simulink model "model_1"  (R2017a)
settings: Solver=VariableStepAuto  StartTime=0.0  StopTime=200000  FixedStep=0.0001  RelTol=1e-6
values from neighbouring files (symbols this model uses):
  c = 3    [Zbiornik.m]
  F_C = Fc0    (= 27)    [Zbiornik.m]
  F_D = Fd0    (= 12)    [Zbiornik.m]
  F_H = Fh0    (= 15)    [Zbiornik.m]
settings Model: Creator=dq  LastModifiedBy=dq

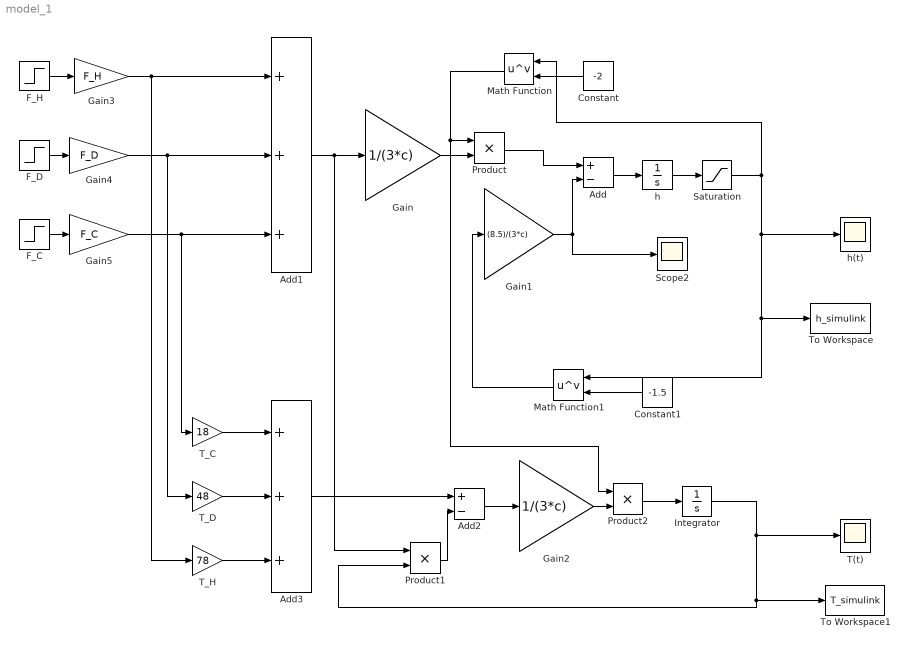
== system model_1 ==
  Add : Sum  Inputs=+-
  Add1 : Sum  Inputs=+++
  Add2 : Sum  Inputs=+-
  Add3 : Sum  Inputs=+++
  Constant : Constant  Value=-2
  Constant1 : Constant  Value=-1.5
  F_C : Step  SampleTime=0
  F_D : Step  SampleTime=0
  F_H : Step  SampleTime=0
  Gain : Gain  Gain=1/(3*c)
  Gain1 : Gain  Gain=(8.5)/(3*c)
  Gain2 : Gain  Gain=1/(3*c)
  Gain3 : Gain  Gain=F_H
  Gain4 : Gain  Gain=F_D
  Gain5 : Gain  Gain=F_C
  Integrator : Integrator
  Math Function : Math  Operator=pow  OutputSignalType=real  SaturateOnIntegerOverflow=on
  Math Function1 : Math  Operator=pow  OutputSignalType=real  SaturateOnIntegerOverflow=on
  Product : Product
  Product1 : Product
  Product2 : Product
  Saturation : Saturate  UpperLimit=5000  LowerLimit=0
  Scope2 : Scope
  T(t) : Scope
  T_C : Gain  Gain=18
  T_D : Gain  Gain=48
  T_H : Gain  Gain=78
  To Workspace : ToWorkspace  VariableName=h_simulink  SaveFormat=Timeseries  SampleTime=-1
  To Workspace1 : ToWorkspace  VariableName=T_simulink  SaveFormat=Timeseries  SampleTime=-1
  h : Integrator  InitialCondition=3
  h(t) : Scope
  wires:
  Add1/1 -> Product1/1, Gain/1
  F_H/1 -> Gain3/1
  Product/1 -> Add/1
  Add/1 -> h/1
  Gain/1 -> Product/2
  Constant/1 -> Math Function/2
  h/1 -> Saturation/1
  Math Function/1 -> Product2/1, Product/1
  Constant1/1 -> Math Function1/2
  Integrator/1 -> Product1/2, To Workspace1/1, T(t)/1
  Add3/1 -> Add2/1
  Product1/1 -> Add2/2
  Add2/1 -> Gain2/1
  Saturation/1 -> Math Function/1, h(t)/1, To Workspace/1, Math Function1/1
  Gain1/1 -> Scope2/1, Add/2
  Gain3/1 -> Add1/1, T_H/1
  F_D/1 -> Gain4/1
  Gain4/1 -> T_D/1, Add1/2
  F_C/1 -> Gain5/1
  Gain5/1 -> T_C/1, Add1/3
  Math Function1/1 -> Gain1/1
  Gain2/1 -> Product2/2
  Product2/1 -> Integrator/1
  T_C/1 -> Add3/1
  T_D/1 -> Add3/2
  T_H/1 -> Add3/3
